simulink model "pole_pairs_id"  (R2023a)
settings: configuration reference "config" (kept outside this file)
libraries: simulink x2
settings Model: DataDictionary=model_config.sldd  Creator=huangcheng  LastModifiedBy=Administrator
settings ConfigSetRef: SourceName=config

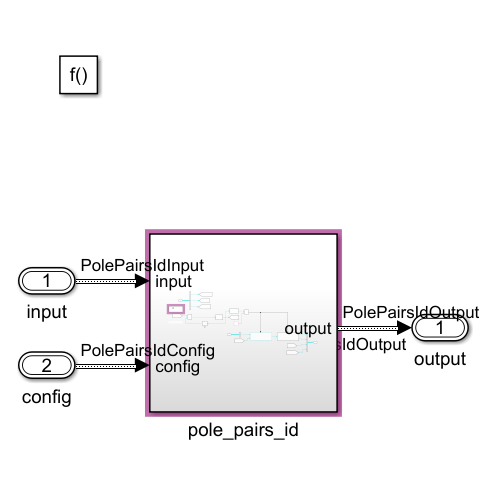
[thumbnail: Simulink's stored preview of the top-level diagram]
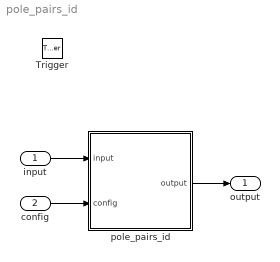
== system pole_pairs_id ==
  input : Inport  OutDataTypeStr=Bus: PolePairsIdInput  BusOutputAsStruct=on
  config : Inport  Port=2  OutDataTypeStr=Bus: PolePairsIdConfig  BusOutputAsStruct=on
  Trigger : TriggerPort  TriggerType=function-call  VariantControl=(inherit)  PortDimensions=1
  pole_pairs_id : Subsystem  SystemSampleTime=10e-5
  output : Outport  OutDataTypeStr=Bus: PolePairsIdOutput  BusOutputAsStruct=on
  wires:
  config/1 -> pole_pairs_id/2(config)
  input/1 -> pole_pairs_id/1(input)
  pole_pairs_id/1(output) -> output/1

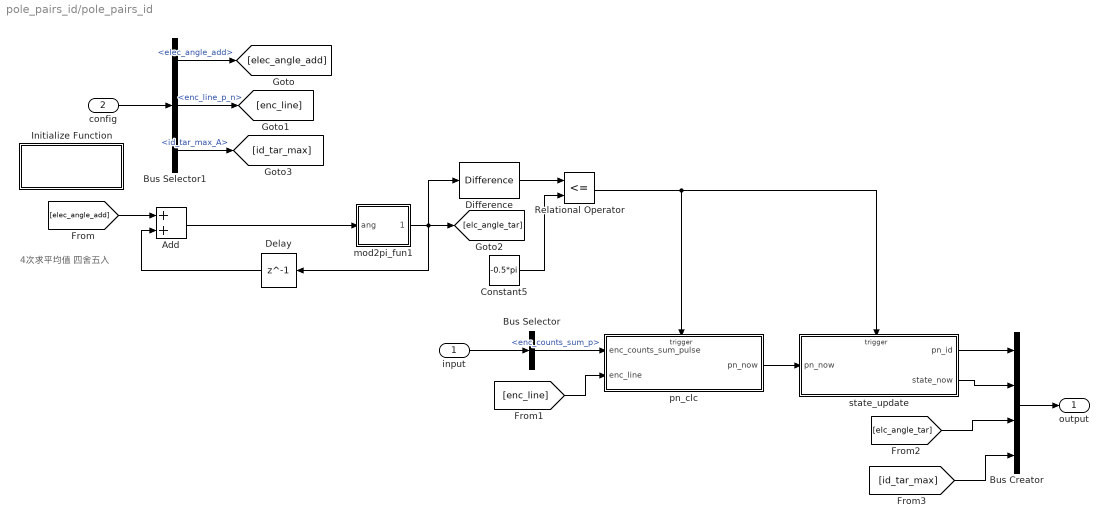
== system pole_pairs_id/pole_pairs_id ==
  note: 4次求平均值 四舍五入
  input : Inport
  config : Inport  Port=2
  Add : Sum
  Bus Creator : BusCreator  Inputs=4  OutDataTypeStr=Bus: PolePairsIdOutput  NonVirtualBus=on
      settings: InheritFromInputs=off
  Bus Selector : BusSelector  OutputSignals=enc_counts_sum_p
  Bus Selector1 : BusSelector  OutputSignals=elec_angle_add,enc_line_p_n,id_tar_max_A
  Constant5 : Constant  Value=-0.5*pi
  Delay : Delay  DelayLength=1  StateName=elec_angle_tar_last
  Difference : simulink/Discrete/Difference  ICPrevInput=0.0  OutMin=[]  OutMax=[]  OutDataType=fixdt(1, 16)  OutScaling=2^-10  DoSatur=off
  Initialize Function : Subsystem  TreatAsAtomicUnit=on
  Relational Operator : RelationalOperator  Operator=<=  OutDataTypeStr=boolean  RndMeth=Simplest  InputSameDT=off
  mod2pi_fun1 : MATLAB Function  TreatAsAtomicUnit=on
  pn_clc : Subsystem
  state_update : Subsystem
  output : Outport
  wires:
  config/1 -> Bus Selector1/1
  Constant5/1 -> Relational Operator/2
  mod2pi_fun1/1(n_ang) -> Difference/1, Delay/1, [elc_angle_tar]
  state_update/2(state_now) -> Bus Creator/2
  Add/1 -> mod2pi_fun1/1(ang)
  Bus Selector1/1 -> [elec_angle_add]  "<elec_angle_add>"
  [elec_angle_add] -> Add/1
  Delay/1 -> Add/2
  Bus Selector1/2 -> [enc_line]  "<enc_line_p_n>"
  Bus Selector1/3 -> [id_tar_max]  "<id_tar_max_A>"
  Difference/1 -> Relational Operator/1
  input/1 -> Bus Selector/1
  state_update/1(pn_id) -> Bus Creator/1
  Bus Selector/1 -> pn_clc/1(enc_counts_sum_pulse)  "<enc_counts_sum_p>"
  [enc_line] -> pn_clc/2(enc_line)
  pn_clc/1(pn_now) -> state_update/1(pn_now)
  [elc_angle_tar] -> Bus Creator/3
  [id_tar_max] -> Bus Creator/4
  Bus Creator/1 -> output/1
  Relational Operator/1 -> pn_clc/Trigger, state_update/Trigger

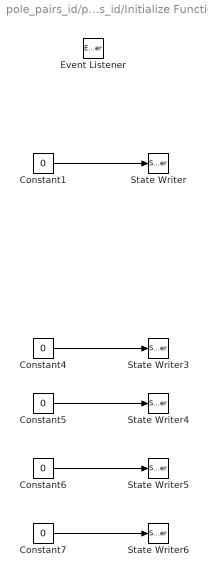
== system pole_pairs_id/pole_pairs_id/Initialize Function ==
  Constant1 : Constant  Value=0  OutDataTypeStr=single
  Constant4 : Constant  Value=0  OutDataTypeStr=boolean
  Constant5 : Constant  Value=0  OutDataTypeStr=uint32
  Constant6 : Constant  Value=0  OutDataTypeStr=uint32
  Constant7 : Constant  Value=0  OutDataTypeStr=uint32
  Event Listener : EventListener  DisableCoverage=on  EventName=reset
  State Writer : StateWriter  StateOwnerBlock=../../Delay  StateName=elec_angle_tar_last
  State Writer3 : StateWriter  StateOwnerBlock=../../pn_clc/Trigger
  State Writer4 : StateWriter  StateOwnerBlock=../../pn_clc/pn_now
  State Writer5 : StateWriter  StateOwnerBlock=../../state_update/Delay  StateName=pn_sum
  State Writer6 : StateWriter  StateOwnerBlock=../../state_update/Delay2  StateName=step_num
  wires:
  Constant1/1 -> State Writer/1
  Constant4/1 -> State Writer3/1
  Constant5/1 -> State Writer4/1
  Constant6/1 -> State Writer5/1
  Constant7/1 -> State Writer6/1

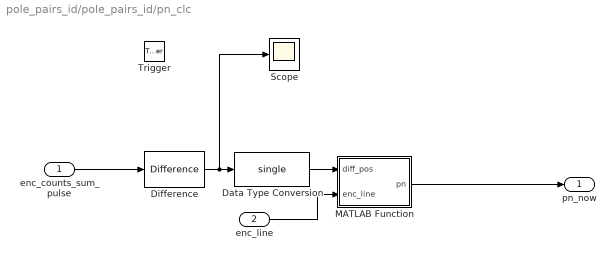
== system pole_pairs_id/pole_pairs_id/pn_clc ==
  enc_counts_sum_pulse : Inport
  enc_line : Inport  Port=2
  Trigger : TriggerPort  VariantControl=(inherit)  PortDimensions=1
  Data Type Conversion : DataTypeConversion  OutDataTypeStr=single  SaturateOnIntegerOverflow=off  RndMeth=Floor
  Difference : simulink/Discrete/Difference  ICPrevInput=0.0  OutMin=[]  OutMax=[]  OutDataType=fixdt(1, 16)  OutScaling=2^-10  DoSatur=off
  MATLAB Function : MATLAB Function  TreatAsAtomicUnit=on
  Scope : Scope
  pn_now : Outport
  wires:
  enc_counts_sum_pulse/1 -> Difference/1
  Difference/1 -> Scope/1, Data Type Conversion/1
  MATLAB Function/1(pn) -> pn_now/1
  enc_line/1 -> MATLAB Function/2(enc_line)
  Data Type Conversion/1 -> MATLAB Function/1(diff_pos)

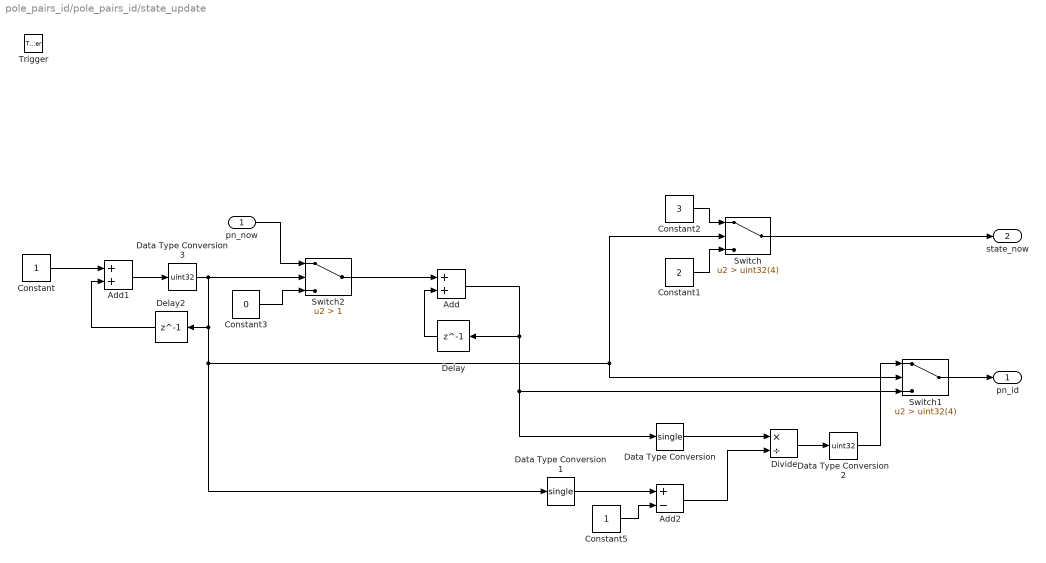
== system pole_pairs_id/pole_pairs_id/state_update ==
  pn_now : Inport
  Trigger : TriggerPort  VariantControl=(inherit)  PortDimensions=1
  Add : Sum
  Add1 : Sum
  Add2 : Sum  Inputs=+-
  Constant : Constant  OutDataTypeStr=uint32
  Constant1 : Constant  Value=2  OutDataTypeStr=int8
  Constant2 : Constant  Value=3  OutDataTypeStr=int8
  Constant3 : Constant  Value=0  OutDataTypeStr=uint32
  Constant5 : Constant  OutDataTypeStr=single
  Data Type Conversion : DataTypeConversion  OutDataTypeStr=single  SaturateOnIntegerOverflow=off  RndMeth=Floor
  Data Type Conversion1 : DataTypeConversion  OutDataTypeStr=single  SaturateOnIntegerOverflow=off  RndMeth=Floor
  Data Type Conversion2 : DataTypeConversion  OutDataTypeStr=uint32  RndMeth=Round  SaturateOnIntegerOverflow=off
  Data Type Conversion3 : DataTypeConversion  OutDataTypeStr=uint32  SaturateOnIntegerOverflow=off  RndMeth=Floor
  Delay : Delay  DelayLength=1  StateName=pn_sum
  Delay2 : Delay  DelayLength=1  InitialCondition=uint32(0)  StateName=step_num
  Divide : Product  Inputs=*/
  Switch : Switch  Criteria=u2 > Threshold  Threshold=uint32(4)  SaturateOnIntegerOverflow=off  InputSameDT=off
  Switch1 : Switch  Criteria=u2 > Threshold  Threshold=uint32(4)  SaturateOnIntegerOverflow=off  InputSameDT=off
  Switch2 : Switch  Criteria=u2 > Threshold  Threshold=1  SaturateOnIntegerOverflow=off  InputSameDT=off
  pn_id : Outport
  state_now : Outport  Port=2
  wires:
  Delay/1 -> Add/2
  Delay2/1 -> Add1/2
  Constant/1 -> Add1/1
  Constant1/1 -> Switch/3
  Constant2/1 -> Switch/1
  Switch/1 -> state_now/1
  Divide/1 -> Data Type Conversion2/1
  Add1/1 -> Data Type Conversion3/1
  Add/1 -> Delay/1, Data Type Conversion/1, Switch1/3
  Data Type Conversion/1 -> Divide/1
  Switch1/1 -> pn_id/1
  Data Type Conversion3/1 -> Data Type Conversion1/1, Switch1/2, Switch/2, Delay2/1, Switch2/2
  Data Type Conversion2/1 -> Switch1/1
  Switch2/1 -> Add/1
  pn_now/1 -> Switch2/1
  Constant3/1 -> Switch2/3
  Data Type Conversion1/1 -> Add2/1
  Add2/1 -> Divide/2
  Constant5/1 -> Add2/2

== matlab function pole_pairs_id/pn_clc/MATLAB Function ==
  data: diff_pos input; pn output; enc_line input
function pn  = direction_id(diff_pos, enc_line)

if diff_pos ~= 0
    pn = uint32(round(single(enc_line) / diff_pos));
else
    pn = uint32(1);
end

== matlab function pole_pairs_id/mod2pi_fun1 ==
  data: ang input; n_ang output
function n_ang = mod2pi(ang)
    % 将角度限制在0到2π范围内
    TWO_PI = single(2*pi);
    n_ang = single(ang);
    while n_ang < 0
        n_ang = n_ang + TWO_PI;
    end
    while n_ang >= TWO_PI
        n_ang = n_ang - TWO_PI;
    end
end
